simulink model "Tavola3_dinamicaF"  (R2018b)
settings: Solver=FixedStepAuto  StartTime=0.0  StopTime=70  RelTol=1e-3
libraries: simulink x1
settings Model: Creator=Utente  LastModifiedBy=giga4

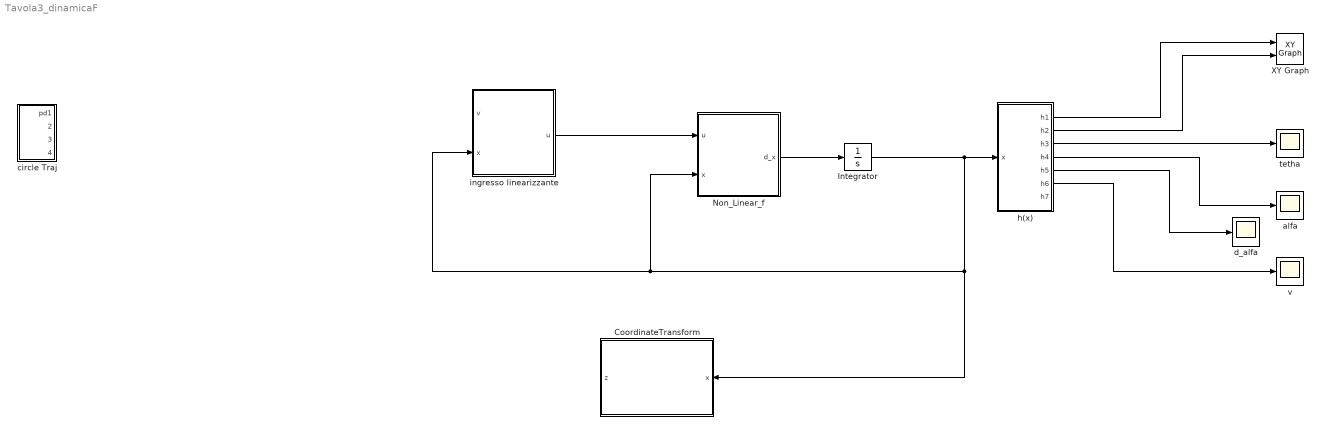
== system Tavola3_dinamicaF ==
  CoordinateTransform : MATLAB Function  TreatAsAtomicUnit=on
  Integrator : Integrator  InitialCondition=[0,0,pi/2,0.017,0,5,0,0]
  "Non_Linear_f " : MATLAB Function  TreatAsAtomicUnit=on
  XY Graph : simulink/Sinks/XY Graph  xmin=-100  xmax=100  ymin=-100  ymax=100  st=-1
  alfa : Scope
  circle Traj : Subsystem
  d_alfa : Scope
  h(x) : MATLAB Function  TreatAsAtomicUnit=on
  ingresso linearizzante : MATLAB Function  TreatAsAtomicUnit=on
  tetha : Scope
  v : Scope
  wires:
  "Non_Linear_f "/1(d_x) -> Integrator/1
  Integrator/1 -> ingresso linearizzante/2(x), "Non_Linear_f "/2(x), CoordinateTransform/1(x), h(x)/1(x)
  ingresso linearizzante/1(u) -> "Non_Linear_f "/1(u)
  h(x)/3(h3) -> tetha/1
  h(x)/4(h4) -> alfa/1
  h(x)/1(h1) -> XY Graph/1
  h(x)/2(h2) -> XY Graph/2
  h(x)/6(h6) -> v/1
  h(x)/5(h5) -> d_alfa/1

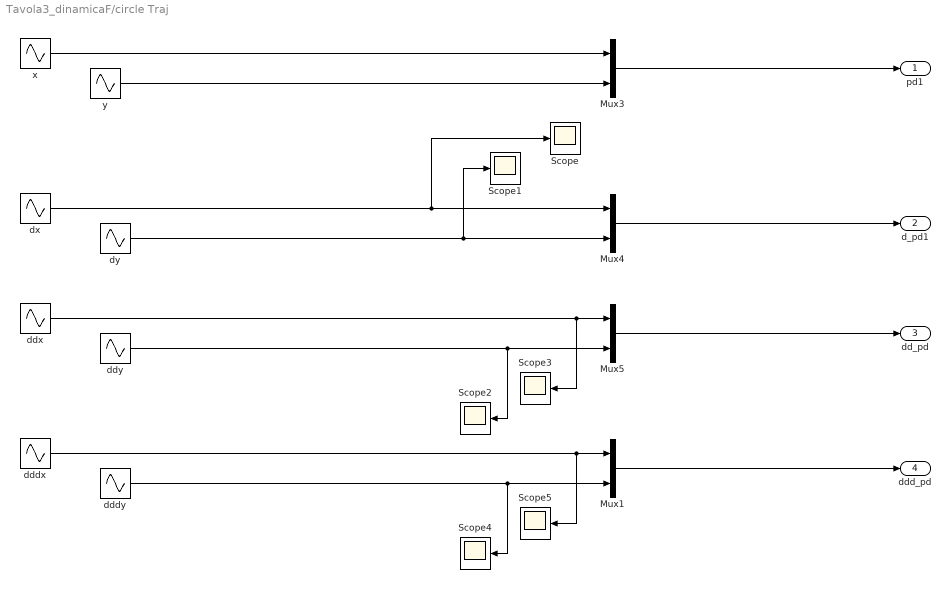
== system Tavola3_dinamicaF/circle Traj ==
  Mux{1,3..5} (4 alike) : Mux  Inputs=2
  Scope{,1..5} (6 alike) : Scope
  dddx : Sin  Amplitude=10  SampleTime=0
  dddy : Sin  Amplitude=-10  Phase=pi/2  SampleTime=0
  ddx : Sin  Amplitude=-10  Phase=pi/2  SampleTime=0
  ddy : Sin  Amplitude=-10  SampleTime=0
  dx : Sin  Amplitude=-10  SampleTime=0
  dy : Sin  Amplitude=10  Phase=pi/2  SampleTime=0
  x : Sin  Amplitude=10  Phase=pi/2  SampleTime=0
  y : Sin  Amplitude=10  SampleTime=0
  pd1 : Outport
  d_pd1 : Outport  Port=2
  dd_pd : Outport  Port=3
  ddd_pd : Outport  Port=4
  wires:
  ddx/1 -> Scope3/1, Mux5/1
  Mux3/1 -> pd1/1
  x/1 -> Mux3/1
  dddy/1 -> Scope4/1, Mux1/2
  ddy/1 -> Scope2/1, Mux5/2
  Mux1/1 -> ddd_pd/1
  dx/1 -> Scope/1, Mux4/1
  dy/1 -> Scope1/1, Mux4/2
  Mux5/1 -> dd_pd/1
  y/1 -> Mux3/2
  dddx/1 -> Scope5/1, Mux1/1
  Mux4/1 -> d_pd1/1

== matlab function Tavola3_dinamicaF/h(x) ==
  data: x input; h1 output; h2 output; h3 output; h4 output; h5 output; h6 output; h7 output
function [h1,h2,h3,h4,h5,h6,h7] = h(x)

x1 = x(1);
x2 = x(2);
x3 = x(3);
x4 = x(4);
x5 = x(5);
x6 = x(6);
x7 = x(7);


h1 = x1;
h2 = x2;
h3 = x3;
h4 = x4;
h5 = x5;
h6 = x6;
h7 = x7;

== matlab function Tavola3_dinamicaF/Non_Linear_f  ==
  data: u input; d_x output; x input
function d_x = statespacef(u,x)

% u è la derivata dell'ingresso è il TauR

x1 = x(1);
x2 = x(2);
x3 = x(3);
x4 = x(4);
x5 = x(5);
x6 = x(6);
x7 = x(7);
x8 = x(8);

f =                                                                                                                              [x6*cos(x3);
                                                                                                                                  x6*sin(x3);
                                                                                                                                          x7;
                                                                                                                                          x5;
 (2.39*sin(2.0*x4)*x5^2)/(4.79*cos(x4)^2 - 12.5) - (173.0*sin(x4))/(4.79*cos(x4)^2 - 12.5) - (3.28*x7^2*sin(2.0*x4))/(4.79*cos(x4)^2 - 12.5);
       (1.99*sin(3.0*x4) - 6.77*sin(x4))*x7^2 + (23.5*sin(2.0*x4))/(4.79*cos(x4)^2 - 12.5) - (2.19*x5^2*sin(2.0*x4))/(4.79*cos(x4)^2 - 12.5);
                                       (0.547*x6*x7*sin(x4))/(0.228*cos(x4)^2 - 0.315) + (0.228*x5*x7*sin(2.0*x4))/(0.228*cos(x4)^2 - 0.315);
                                                                                                                                          0];

g1 = [                                              0;
                                                    0;
                                                    0;
                                                    0;
        (2.19*cos(x3) + 3.11)/(4.79*cos(x4)^2 - 12.5);
 -(1.0*(0.547*cos(x4) + 1.0))/(4.79*cos(x4)^2 - 12.5);
                      -0.05/(0.228*cos(x4)^2 - 0.315);
                                                   0];
                                               
f_tilde = [f+g1*x8]         

g1_tilde = [0;0;0;0;0;0;0;1];
    
g2 = [                                              0;
                                                    0;
                                                    0;
                                                    0;
        (2.19*cos(x3) + 3.11)/(4.79*cos(x4)^2 - 12.5);
 -(1.0*(0.547*cos(x4) + 1.0))/(4.79*cos(x4)^2 - 12.5);
                       0.05/(0.228*cos(x4)^2 - 0.315);
                                                   0];
d_x = f_tilde + [g1_tilde,g2]*u;

== matlab function Tavola3_dinamicaF/ingresso linearizzante ==
  data: v input; u output; x input
function u = inputLinearizzante(v,x)

x1 = x(1);
x2 = x(2);
x3 = x(3);
x4 = x(4);
x5 = x(5);
x6 = x(6);
x7 = x(7);
x8 = x(8);



 
 u = -inv_E*Gamma+inv_E*v;

== matlab function Tavola3_dinamicaF/CoordinateTransform ==
  data: z output; x input
function z = transformCoordinate(x)

x1 = x(1);
x2 = x(2);
x3 = x(3);
x4 = x(4);
x5 = x(5);
x6 = x(6);
x7 = x(7);
x8 = x(8);

z =    [                                                                                                                                                      x1;
                                                                                                                                                      x6*cos(x3);
 cos(x3)*((1.99*sin(3.0*x4) - 6.77*sin(x4))*x7^2 + (23.5*sin(2.0*x4))/(4.79*cos(x4)^2 - 12.5) - (2.19*x5^2*sin(2.0*x4))/(4.79*cos(x4)^2 - 12.5)) - x6*x7*sin(x3);
                                                                                                                                                              x2;
                                                                                                                                                      x6*sin(x3);
 sin(x3)*((1.99*sin(3.0*x4) - 6.77*sin(x4))*x7^2 + (23.5*sin(2.0*x4))/(4.79*cos(x4)^2 - 12.5) - (2.19*x5^2*sin(2.0*x4))/(4.79*cos(x4)^2 - 12.5)) + x6*x7*cos(x3);
                                                                                                                                                              x5;
                                                                                                                                                              x7];
